simulink model "pcb_heating_ControlLoop"  (R2024a)
settings: Solver=ode15s  StartTime=0.0  StopTime=2500  RelTol=1e-3
values from neighbouring files (symbols this model uses):
  A = [-1/(C_L*R_h)-1/(C_L*R_cond),   1/(C_L*R_cond) ... (first row only)    [initTemperatureControl.m]    (also in pcb_heating_statespace.m = [ -(1/R_h + 1/R_cond)/C_L,    ( 1/R_cond )/C_L)
  B = [1/C_L; 0]    [initTemperatureControl.m]    (also in pcb_heating_statespace.m = [ 1/C_L ; 0 ])
  C = eye(2)    [initTemperatureControl.m]    (also in pcb_heating_statespace.m)
  D = [0; 0]    [initTemperatureControl.m]    (also in pcb_heating_statespace.m = zeros(2,1))
  ss_L = minreal( ss(sys_L) )    [pcb_identify_tf_and_plot.m]
  ss_R = minreal( ss(sys_R) )    [pcb_identify_tf_and_plot.m]
libraries: slpidlib x6
settings Model: Creator=arkad  LastModifiedBy=arkad

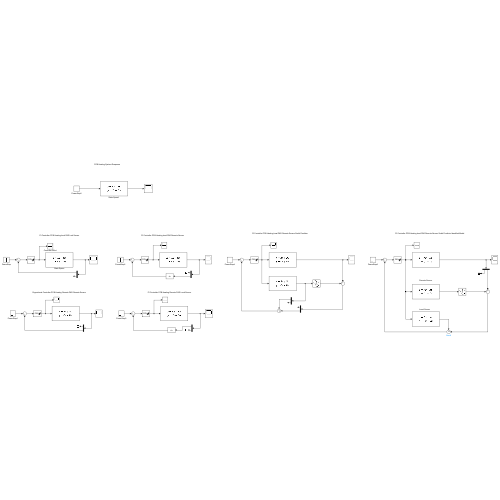
[thumbnail: Simulink's stored preview of the top-level diagram]
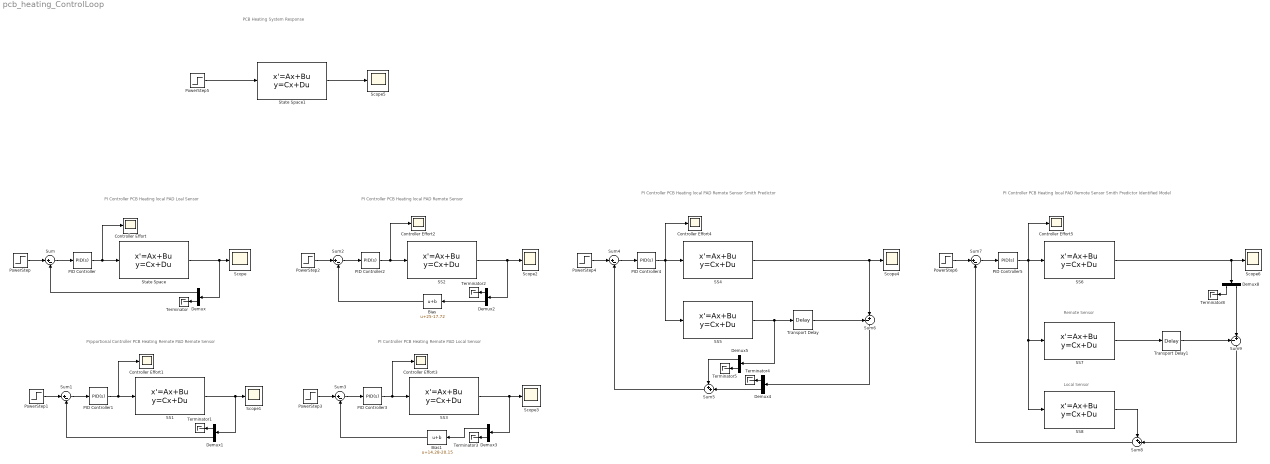
== system pcb_heating_ControlLoop ==
  note: Remote Sensor
  note: PI Controller PCB Heating local PAD Loal Sensor
  note: Prpportional Controller PCB Heating Remote PAD Remote Sensor
  note: PI Controller PCB Heating local PAD Remote Sensor
  note: PI Controller PCB Heating Remote PAD Local Sensor
  note: PI Controller PCB Heating local PAD Remote Sensor Smith Predictor
  note: PCB Heating System Response
  note: PI Controller PCB Heating local PAD Remote Sensor Smith Predictor Identified Model
  note: Local Sensor
  Bias : Bias  Bias=25-17.72  SaturateOnIntegerOverflow=off
  Bias1 : Bias  Bias=14.28-20.15  SaturateOnIntegerOverflow=off
  Controller Effort{,1..5} (6 alike) : Scope
  Demux{,1..5,8} (7 alike) : Demux  Outputs=2
  PID Controller{,1..5} (6 alike) : slpidlib/PID Controller  Controller=PID  Form=Parallel  TimeDomain=Continuous-time  UseExternalTs=off  SampleTime=-1  IntegratorMethod=Forward Euler  FilterMethod=Forward Euler  ControllerParametersSource=internal  P=1  I=0.01  UseKiTs=off  D=0  UseExternalDerivativeSource=off  N=100  UseFilter=on  TunerSelectOption=Transfer Function Based (PID Tuner App)  InitialConditionSource=internal  InitialConditionForIntegrator=0  InitialConditionForFilter=0  DifferentiatorICPrevScaledInput=0  ExternalReset=none  TrackingMode=off  Kt=1  LimitOutput=on  SatLimitsSource=internal  UpperSaturationLimit=2.3  LowerSaturationLimit=-2.3  LinearizeAsGain=on  AntiWindupMode=none  Kb=1  LimitIntegrator=on  UpperIntegratorSaturationLimit=2  LowerIntegratorSaturationLimit=-2  POutMin=[]  POutMax=[]  IOutMin=[]  IOutMax=[]  DOutMin=[]  DOutMax=[]  NOutMin=[]  NOutMax=[]  SumOutMin=[]  SumOutMax=[]  SaturationOutMin=[]  SaturationOutMax=[]  PParamMin=[]  PParamMax=[]  IParamMin=[]  IParamMax=[]  DParamMin=[]  DParamMax=[]  NParamMin=[]  NParamMax=[]  KbParamMin=[]  KbParamMax=[]  KtParamMin=[]  KtParamMax=[]  KbOutMin=[]  KbOutMax=[]  KtOutMin=[]  KtOutMax=[]  IntegratorOutMin=[]  IntegratorOutMax=[]  FilterOutMin=[]  FilterOutMax=[]  SumI1OutMin=[]  SumI1OutMax=[]  SumI2OutMin=[]  SumI2OutMax=[]  SumI3OutMin=[]  SumI3OutMax=[]  SumI4OutMin=[]  SumI4OutMax=[]  SumDOutMin=[]  SumDOutMax=[]  DifferentiatorOutMin=[]  DifferentiatorOutMax=[]  FilterDiffOutCoefMin=[]  FilterDiffOutCoefMax=[]  ReciprocalOutMin=[]  ReciprocalOutMax=[]  SumDenOutMin=[]  SumDenOutMax=[]  SumNumOutMin=[]  SumNumOutMax=[]  DivideOutMin=[]  DivideOutMax=[]  UdiffTsProdOutMin=[]  UdiffTsProdOutMax=[]  NTsProdOutMin=[]  NTsProdOutMax=[]  UintegralTsProdOutMin=[]  UintegralTsProdOutMax=[]  UngainTsProdOutMin=[]  UngainTsProdOutMax=[]  ClampingZeroOutDataTypeStr=Inherit: Inherit via back propagation  ClampingZeroOutMin=[]  ClampingZeroOutMax=[]  FilterDenConstantOutDataTypeStr=Inherit: Inherit via back propagation  FilterDenConstantOutMin=[]  FilterDenConstantOutMax=[]  PCopyOutDataTypeStr=Inherit: Inherit via back propagation  PCopyOutMin=[]  PCopyOutMax=[]  NCopyOutDataTypeStr=Inherit: Inherit via back propagation  NCopyOutMin=[]  NCopyOutMax=[]  IntegratorContinuousStateAttributes=''  IntegratorStateMustResolveToSignalObject=off  IntegratorRTWStateStorageClass=Auto  FilterContinuousStateAttributes=''  FilterStateMustResolveToSignalObject=off  FilterRTWStateStorageClass=Auto  ParallelPVariant=InternalParameters  IdealPVariant=Disabled  IVariant=InternalParameters  DVariant=InternalParameters  IntegratorVariant=Continuous  SatVariant=Enabled  AWVariant=Passthrough  PCopyVariant=Disabled  TRVariant=Disabled  FdbkBlocksVariant=Forward  IdealPFdbkVariant=Disabled  SatFdbkVariant=Disabled  DerivativeFilterVariant=ContFilter  NVariant=InternalParameters  NCopyVariant=Disabled  FilterICVariant=InternalICsFilter  IntegratorICVariant=InternalICs  ExternalResetVariant=Disabled  TRSumVariant=Passthrough  SumFdbkVariant=Disabled  SumVariant=Sum_PID  TsampFilterVariant=InternalTs  TsampNgainVariant=Passthrough  TsampIntegralVariant=Disabled_SignalSpec  ExternalSaturationOutDataTypeStr=Inherit: Same as second input  DerivativeSourceVariant=ErrorSignal
  PowerStep{,2,4,6} (4 alike) : Step  Time=0  After=25  SampleTime=0
  PowerStep1 : Step  Time=0  After=15  SampleTime=0
  PowerStep3 : Step  Time=0  After=15  SampleTime=0
  PowerStep5 : Step  Time=0  SampleTime=0
  SS{1..6} (6 alike) : StateSpace  A=A  B=B  C=C  D=D  InitialCondition=0
  SS7 : StateSpace  A=ss_R.A  B=ss_R.B  C=ss_R.C  D=ss_R.D  InitialCondition=0
  SS8 : StateSpace  A=ss_L.A  B=ss_L.B  C=ss_L.C  D=ss_L.D  InitialCondition=0
  Scope{,1..6} (7 alike) : Scope
  State Space : StateSpace  A=A  B=B  C=C  D=D  InitialCondition=0
  State Space1 : StateSpace  A=A  B=B  C=C  D=D  InitialCondition=0
  Sum{,1..4,7} (6 alike) : Sum  Inputs=|+-
  Sum5 : Sum  Inputs=++|
  Sum6 : Sum  Inputs=-+|
  Sum8 : Sum  Inputs=++|
  Sum9 : Sum  Inputs=-+|
  Terminator{,1..5,8} (7 alike) : Terminator
  Transport Delay : TransportDelay  DelayTime=44.0
  Transport Delay1 : TransportDelay  DelayTime=44.0
  wires:
  State Space/1 -> Demux/1, Scope/1
  PowerStep/1 -> Sum/1
  Demux/2 -> Terminator/1
  Sum/1 -> PID Controller/1
  PID Controller/1 -> Controller Effort/1, State Space/1
  Demux/1 -> Sum/2
  PID Controller1/1 -> Controller Effort1/1, SS1/1
  PowerStep1/1 -> Sum1/1
  Sum1/1 -> PID Controller1/1
  SS1/1 -> Demux1/1, Scope1/1
  Demux1/1 -> Terminator1/1
  Demux1/2 -> Sum1/2
  PID Controller2/1 -> Controller Effort2/1, SS2/1
  PowerStep2/1 -> Sum2/1
  Sum2/1 -> PID Controller2/1
  SS2/1 -> Demux2/1, Scope2/1
  Demux2/1 -> Terminator2/1
  Demux2/2 -> Bias/1
  Bias/1 -> Sum2/2
  PID Controller3/1 -> Controller Effort3/1, SS3/1
  PowerStep3/1 -> Sum3/1
  Sum3/1 -> PID Controller3/1
  SS3/1 -> Demux3/1, Scope3/1
  Bias1/1 -> Sum3/2
  Demux3/2 -> Terminator3/1
  Demux3/1 -> Bias1/1
  Demux4/1 -> Terminator4/1
  Demux4/2 -> Sum5/2
  PowerStep4/1 -> Sum4/1
  Sum4/1 -> PID Controller4/1
  SS4/1 -> Scope4/1, Sum6/2
  PID Controller4/1 -> SS4/1, Controller Effort4/1, SS5/1
  Sum5/1 -> Sum4/2
  SS5/1 -> Transport Delay/1, Demux5/1
  Demux5/1 -> Sum5/1
  Demux5/2 -> Terminator5/1
  Sum6/1 -> Demux4/1
  Transport Delay/1 -> Sum6/1
  PowerStep5/1 -> State Space1/1
  State Space1/1 -> Scope5/1
  Sum8/1 -> Sum7/2
  Sum7/1 -> PID Controller5/1
  PID Controller5/1 -> SS8/1, SS7/1, SS6/1, Controller Effort5/1
  Transport Delay1/1 -> Sum9/1
  PowerStep6/1 -> Sum7/1
  SS6/1 -> Scope6/1, Demux8/1
  Demux8/1 -> Terminator8/1
  Demux8/2 -> Sum9/2
  Sum9/1 -> Sum8/2
  SS7/1 -> Transport Delay1/1
  SS8/1 -> Sum8/1
